simulink model "assignment3_M_T"  (R2012b)
settings: Solver=ode45  StartTime=0.0  StopTime=210  RelTol=1e-3
undefined symbols (not defined in the file): mfs, rls
libraries: simulink x1
CloseFcn:
  | rtwprivate ssgensfun ModelCloseRequest nlgentpl
settings Model: ExtModeAutoUpdateStatusClock=off  BufferReuse=off  Creator=lbusoniu  LastModifiedBy=stnavalkar
settings DataIOCC: SignalLoggingSaveFormat=ModelDataLogs  SaveOutput=off  SaveTime=off  SignalLoggingName=sigsOut
settings OptimizationCC: OptimizeBlockIOStorage=off  BufferReuse=off  ExpressionFolding=off  ExpressionDepthLimit=128  LocalBlockOutputs=off  InitFltsAndDblsToZero=on
settings DebuggingCC: SaveWithParameterizedLinksMsg=none  SignalResolutionControl=TryResolveAllWithWarning  SolverPrmCheckMsg=none  MultiTaskDSMMsg=warning  MultiTaskCondExecSysMsg=none  FcnCallInpInsideContextMsg=UseLocalSettings  StateNameClashWarn=none  StrictBusMsg=None
settings HardwareCC: TargetUnknown=on
settings RTWCC: IncludeERTFirstTime=on
settings CodeAppCC: CustomSymbolStrType=$N$R$M_T  InternalIdentifier=Shortened
settings GRTTargetCC: TargetFcnLib=ansi_tfl_tmw.mat  CodeReplacementLibrary=None  CombineOutputUpdateFcns=off  CPPClassGenCompliant=on  GRTInterface=on

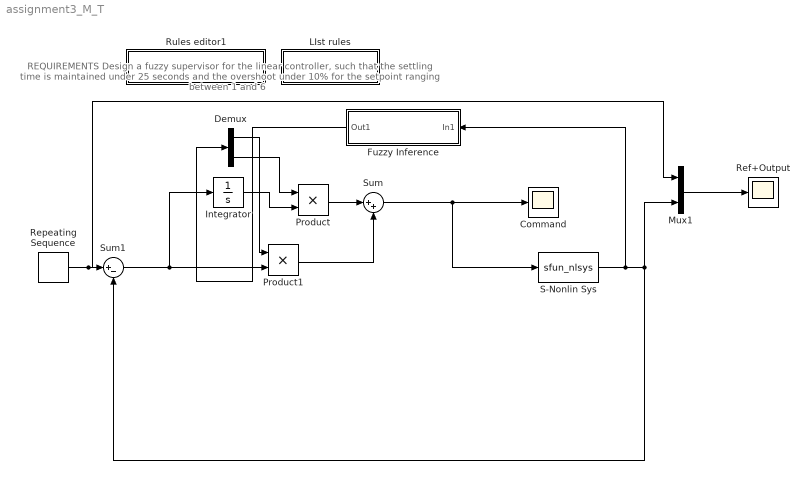
== system assignment3_M_T ==
  note: REQUIREMENTS
      | Design a fuzzy supervisor for the linear controller, such that
      | the settling time is maintained under 25 seconds and the overshoot under 10%
      | for the setpoint ranging between 1 and 6
  Command : Scope
      settings: TimeRange=250  YMin=-0.2  YMax=0.2  SaveName=u
  Demux : Demux  Outputs=2
  Fuzzy Inference : Subsystem  mask(Fuzzy inference block){rls=rls, mfs=mfs, def=[1 3]}
      mask prompts: rls "Rule matrix:"; mfs "Membership functions matrix:"; def "Default output:"
      mask help:
      | MIN-MAX inference with
      |  fuzzy means defuzzification
      mask Help: Fuzzy inference block can be used as a direct fuzzy controller or as a fuzzy supervisor. For details on dialog parameters see INFER.
      mask Display: disp('Fuzzy Inference')
  Integrator : Integrator
  LIst rules : Subsystem
      settings: OpenFcn=disp(rls2txt(rls, mfs, inputs, outputs, nlab, labels));
      mask Display: disp('List Fuzzy Rules')
  Mux1 : Mux  Inputs=2
  Product : Product
  Product1 : Product
  Ref+Output : Scope
      settings: TimeRange=250  YMin=1  YMax=7  SaveName=u2
  Repeating Sequence : simulink/Sources/Repeating Sequence  rep_seq_t=[0 30 30.5 60 60.5 90 90.5 120 120.5 150 150.5 180 180.5 211]  rep_seq_y=[4 4 1 1 3 3 2 2 5 5 3 3 6 6]
  Rules editor1 : Subsystem  mask(Rule-base editor){}
      settings: OpenFcn=eval(['[rls, mfs, inputs, outputs, nlab, labels] = txt2rls(''rulebase.rb'');']);
      mask Display: disp('Compile Rulebase')
  S-Nonlin Sys : S-Function  FunctionName=sfun_nlsys  EnableBusSupport=off
  Sum : Sum  Inputs=|++
  Sum1 : Sum  Inputs=|+-  SaturateOnIntegerOverflow=on
  wires:
  Sum1/1 -> Integrator/1, Product1/2
  Sum/1 -> S-Nonlin Sys/1, Command/1
  Mux1/1 -> Ref+Output/1
  Repeating Sequence/1 -> Mux1/1, Sum1/1
  Integrator/1 -> Product/2
  Fuzzy Inference/1(Out1) -> Demux/1
  Demux/1 -> Product1/1
  Demux/2 -> Product/1
  Product1/1 -> Sum/2
  Product/1 -> Sum/1
  S-Nonlin Sys/1 -> Fuzzy Inference/1(In1), Sum1/2, Mux1/2

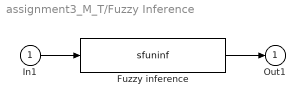
== system assignment3_M_T/Fuzzy Inference ==
  In1 : Inport
  Fuzzy inference : S-Function  FunctionName=sfuninf  Parameters=rls, mfs, def  EnableBusSupport=off
  Out1 : Outport
  wires:
  In1/1 -> Fuzzy inference/1
  Fuzzy inference/1 -> Out1/1

== system assignment3_M_T/LIst rules ==

== system assignment3_M_T/Rules editor1 ==
